simulink model "Amplitude_Ud_Uq"  (R2023a)
settings: Solver=VariableStepAuto  StartTime=0.0  StopTime=2/f  MaxStep=1e-5  RelTol=1e-3
undefined symbols (not defined in the file): E, f
libraries: eeTransforms x1
settings Model: Creator=dougl  LastModifiedBy=dougl

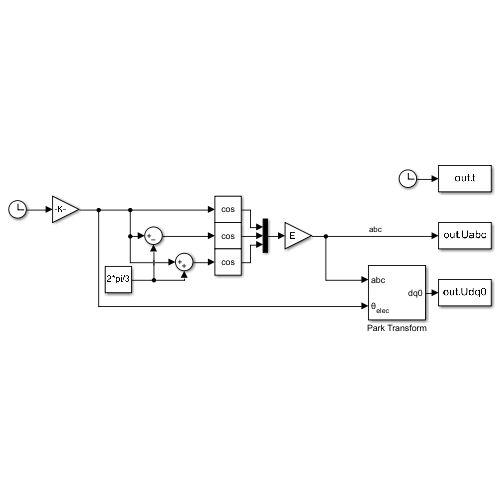
[thumbnail: Simulink's stored preview of the top-level diagram]
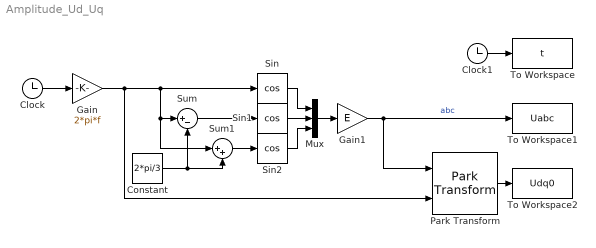
== system Amplitude_Ud_Uq ==
  Clock : Clock
  Clock1 : Clock
  Constant : Constant  Value=2*pi/3
  Gain : Gain  Gain=2*pi*f
  Gain1 : Gain  Gain=E
  Mux : Mux  Inputs=3
  Park Transform : eeTransforms/Park Transform  AxisAlignment=D-axis  PowerInvariant=off
      settings: LibrarySourceBlock=|
      | ee_sl_lib/Mathematical
      | Transforms/Park Transform
  Sin : Trigonometry  Operator=cos
  Sin1 : Trigonometry  Operator=cos
  Sin2 : Trigonometry  Operator=cos
  Sum : Sum  Inputs=|+-
  Sum1 : Sum  Inputs=|++
  To Workspace : ToWorkspace  VariableName=t  SampleTime=-1
  To Workspace1 : ToWorkspace  VariableName=Uabc  SampleTime=-1
  To Workspace2 : ToWorkspace  VariableName=Udq0  SampleTime=-1
  wires:
  Sum/1 -> Sin1/1
  Sum1/1 -> Sin2/1
  Clock/1 -> Gain/1
  Constant/1 -> Sum1/2, Sum/2
  Sin/1 -> Mux/1
  Sin1/1 -> Mux/2
  Sin2/1 -> Mux/3
  Gain1/1 -> To Workspace1/1, Park Transform/1  "abc"
  Gain/1 -> Park Transform/2, Sin/1, Sum1/1, Sum/1
  Clock1/1 -> To Workspace/1
  Park Transform/1 -> To Workspace2/1
  Mux/1 -> Gain1/1
